simulink model "Parte_c_sec_f_sim"  (R2023b)
settings: Solver=VariableStepAuto  StartTime=0.0  StopTime=8  RelTol=1e-3
undefined symbols (not defined in the file): bat_awu_den, bat_awu_num, C_L, cell_awu_den, cell_awu_num, k_bat_inf, k_cell_inf
settings Model: Creator=Admin  LastModifiedBy=gonza
settings ModelReferenceCC: EnableRefExpFcnMdlSchedulingChecks=on

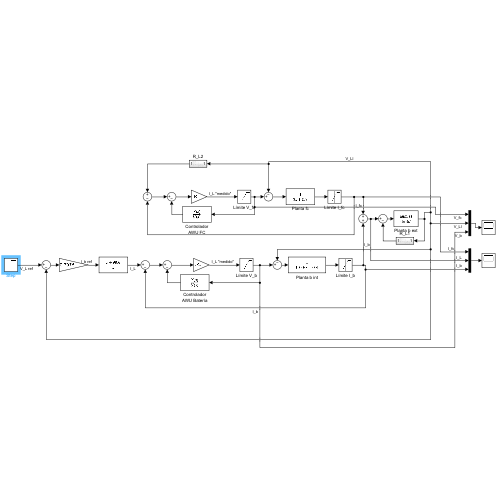
[thumbnail: Simulink's stored preview of the top-level diagram]
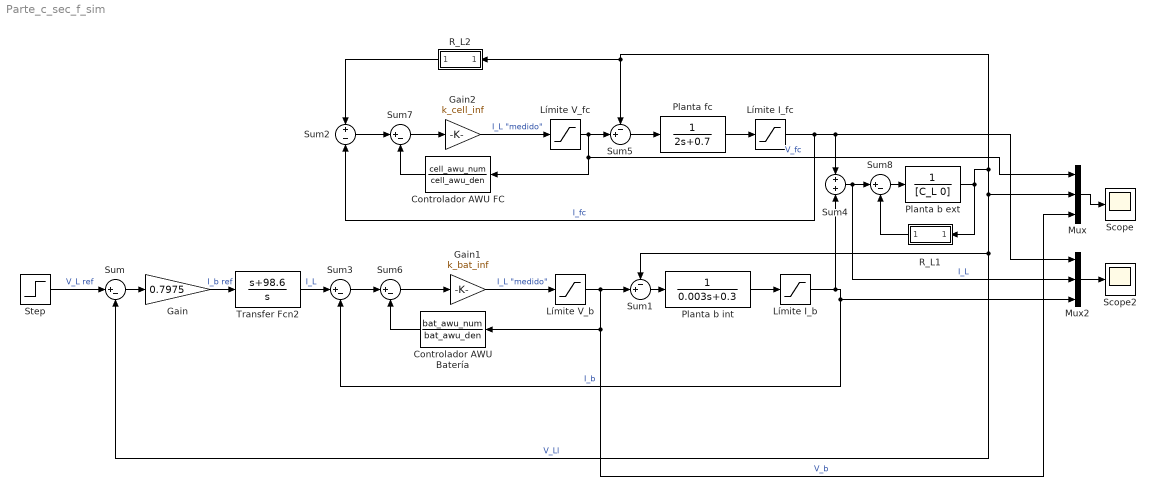
== system Parte_c_sec_f_sim ==
  Controlador AWU Batería : TransferFcn  Numerator=bat_awu_num  Denominator=bat_awu_den
  Controlador AWU FC : TransferFcn  Numerator=cell_awu_num  Denominator=cell_awu_den
  Gain : Gain  Gain=0.7975
  Gain1 : Gain  Gain=k_bat_inf
  Gain2 : Gain  Gain=k_cell_inf
  Límite I_b : Saturate  UpperLimit=120  LowerLimit=-120
  Límite I_fc : Saturate  UpperLimit=200  LowerLimit=0
  Límite V_b : Saturate  UpperLimit=400  LowerLimit=-400
  Límite V_fc : Saturate  UpperLimit=450  LowerLimit=0
  Mux : Mux  Inputs=3
  Mux2 : Mux  Inputs=3
  Planta b ext : TransferFcn  Numerator=1  Denominator=[C_L 0]
  Planta b int : TransferFcn  Denominator=[0.003 0.3]
  Planta fc : TransferFcn  Denominator=[2 0.7]
  R_L1 : Subsystem
  R_L2 : Subsystem
  Scope : Scope
  Scope2 : Scope
  Step : Step  Time=0.1  After=250  SampleTime=0
  Sum{,3,6..8} (5 alike) : Sum  Inputs=|+-
  Sum1 : Sum  Inputs=-+|
  Sum2 : Sum  Inputs=+|-
  Sum4 : Sum  Inputs=+|+
  Sum5 : Sum  Inputs=-+|
  Transfer Fcn2 : TransferFcn  Numerator=[1 98.6]  Denominator=[1 0]
  wires:
  Step/1 -> Sum/1  "V_L ref"
  Transfer Fcn2/1 -> Sum3/1  "I_L"
  Planta b ext/1 -> Sum1/1, Sum/2, Mux/2, R_L2/1(In1), Sum5/1, R_L1/1(In1)  "V_Ll"
  Mux/1 -> Scope/1
  Límite I_b/1 -> Sum3/2, Mux2/3, Sum4/2  "I_b"
  Límite I_fc/1 -> Mux2/1, Sum4/1, Sum2/2  "I_fc"
  Planta b int/1 -> Límite I_b/1
  Planta fc/1 -> Límite I_fc/1
  Límite V_b/1 -> Mux/3, Controlador AWU Batería/1, Sum1/2  "V_b"
  Sum1/1 -> Planta b int/1
  Límite V_fc/1 -> Controlador AWU FC/1, Mux/1, Sum5/2  "V_fc"
  Sum5/1 -> Planta fc/1
  Mux2/1 -> Scope2/1
  Sum6/1 -> Gain1/1
  Controlador AWU Batería/1 -> Sum6/2
  Gain1/1 -> Límite V_b/1  "I_L \"medido\""
  Sum3/1 -> Sum6/1
  Controlador AWU FC/1 -> Sum7/2
  Sum7/1 -> Gain2/1
  Gain2/1 -> Límite V_fc/1  "I_L \"medido\""
  Sum2/1 -> Sum7/1
  Sum/1 -> Gain/1
  Gain/1 -> Transfer Fcn2/1  "I_b ref"
  R_L2/1(Out1) -> Sum2/1
  Sum8/1 -> Planta b ext/1
  R_L1/1(Out1) -> Sum8/2
  Sum4/1 -> Mux2/2, Sum8/1  "I_L"

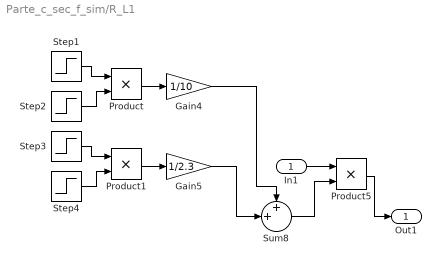
== system Parte_c_sec_f_sim/R_L1 ==
  In1 : Inport
  Gain4 : Gain  Gain=1/10
  Gain5 : Gain  Gain=1/2.3
  Product : Product
  Product1 : Product
  Product5 : Product
  Step1 : Step  Time=0.1  SampleTime=0
  Step2 : Step  Time=2.1  Before=1  After=0  SampleTime=0
  Step3 : Step  Time=2.1  SampleTime=0
  Step4 : Step  Time=5.1  Before=1  After=0  SampleTime=0
  Sum8 : Sum  Inputs=++|
  Out1 : Outport
  wires:
  Step2/1 -> Product/2
  Step3/1 -> Product1/1
  Product/1 -> Gain4/1
  Step4/1 -> Product1/2
  Product1/1 -> Gain5/1
  Gain4/1 -> Sum8/1
  Step1/1 -> Product/1
  Gain5/1 -> Sum8/2
  Product5/1 -> Out1/1
  In1/1 -> Product5/1
  Sum8/1 -> Product5/2

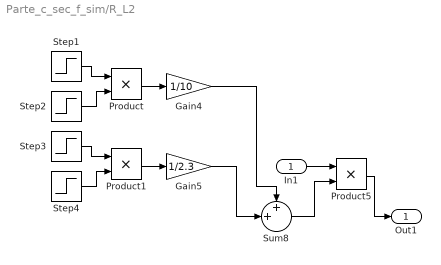
== system Parte_c_sec_f_sim/R_L2 ==
  In1 : Inport
  Gain4 : Gain  Gain=1/10
  Gain5 : Gain  Gain=1/2.3
  Product : Product
  Product1 : Product
  Product5 : Product
  Step1 : Step  Time=0.1  SampleTime=0
  Step2 : Step  Time=2.1  Before=1  After=0  SampleTime=0
  Step3 : Step  Time=2.1  SampleTime=0
  Step4 : Step  Time=5.1  Before=1  After=0  SampleTime=0
  Sum8 : Sum  Inputs=++|
  Out1 : Outport
  wires:
  Step2/1 -> Product/2
  Step3/1 -> Product1/1
  Product/1 -> Gain4/1
  Step4/1 -> Product1/2
  Product1/1 -> Gain5/1
  Gain4/1 -> Sum8/1
  Step1/1 -> Product/1
  Gain5/1 -> Sum8/2
  Product5/1 -> Out1/1
  In1/1 -> Product5/1
  Sum8/1 -> Product5/2
